simulink subsystem "ElectricMachine2"  (R2025b)
settings: Solver=VariableStepAuto  StartTime=0.0  StopTime=10.0  RelTol=1e-3
libraries: autolibmappedmotor x2
settings Model: ModifiedByFormat=The MathWorks, Inc.  Creator=The MathWorks, Inc.  LastModifiedBy=The MathWorks, Inc.
settings SolverCC: MaxZcPerStep=1.0
settings DebuggingCC: UnconnectedInputMsg=warning  UnconnectedOutputMsg=warning  UnconnectedLineMsg=warning
settings ModelReferenceCC: EnableRefExpFcnMdlSchedulingChecks=on
settings RTWCC: GPUComputeCapability=3.5  DLArmComputeVersion=19.05

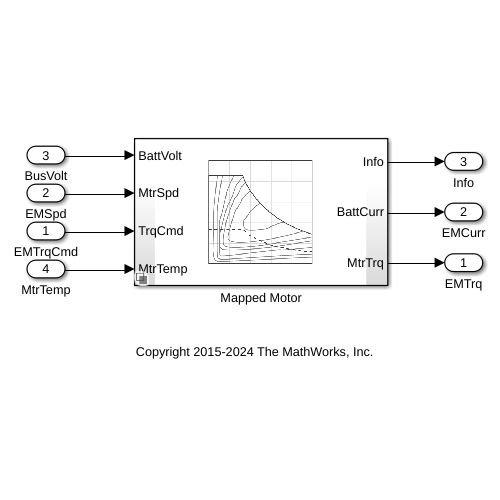
[thumbnail: Simulink's stored preview of the top-level diagram]
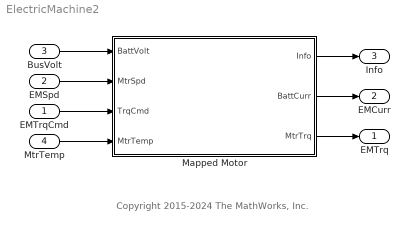
== system ElectricMachine2 ==
  note: Copyright 2015-2024 The MathWorks, Inc.
  EMTrqCmd : Inport
  EMSpd : Inport  Port=2
  BusVolt : Inport  Port=3
  MtrTemp : Inport  Port=4
  Mapped Motor : Subsystem  Variant=on  VariantControlMode=label  LabelModeActiveChoice=MappedMotorCalibrationImport
  EMTrq : Outport  VectorParamsAs1DForOutWhenUnconnected=off
  EMCurr : Outport  Port=2  VectorParamsAs1DForOutWhenUnconnected=off
  Info : Outport  Port=3
  wires:
  EMTrqCmd/1 -> Mapped Motor/3(TrqCmd)
  BusVolt/1 -> Mapped Motor/1(BattVolt)
  EMSpd/1 -> Mapped Motor/2(MtrSpd)
  Mapped Motor/2(BattCurr) -> EMCurr/1
  Mapped Motor/1(Info) -> Info/1
  Mapped Motor/3(MtrTrq) -> EMTrq/1
  MtrTemp/1 -> Mapped Motor/4(MtrTemp)

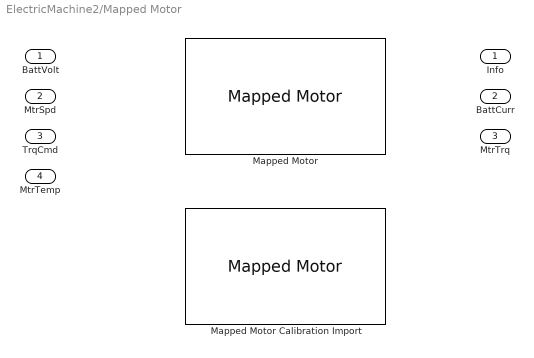
== system ElectricMachine2/Mapped Motor ==
  BattVolt : Inport
  MtrSpd : Inport  Port=2
  TrqCmd : Inport  Port=3
  MtrTemp : Inport  Port=4
  Mapped Motor : autolibmappedmotor/Mapped Motor  VariantControl=MappedMotor  w_Tmax_bp_ext=w_Tmax_bp  Tmax_w_V_ext=Tmax_w_V  w_Tmin_bp_ext=w_Tmin_bp  Tmin_w_V_ext=Tmin_w_V  port_config=Speed  param_by=Tabulated torque-speed envelope  w_t=PlntEM2Spd  T_t=PlntEM2Trq  torque_max=0.1  power_max=30  SpreadsheetTqLimitsFileName=MotorCalibrationImportData.xlsx  Tmax_w_V=PlntEM1MaxTqTbl  w_Tmax_bp=PlntEM1MaxTqSpdBpt  V_Tmax_bp=PlntEM1MaxTqVoltBpt  Tmin_w_V=PlntEM1MinTqTbl  w_Tmin_bp=PlntEM1MinTqSpdBpt  V_Tmin_bp=PlntEM1MinTqVoltBpt  Tc=PlntEM2TimeCnst  param_loss=Tabulated efficiency data  SpreadsheetLossFileName=MotorCalibrationImportData.xlsx  SpreadsheetEffFileName=MotorCalibrationImportData.xlsx  eff=100  w_eff=375  T_eff=0.08  Piron=0  Pbase=0  w_eff_bp=PlntEM2SpdEff  T_eff_bp=PlntEM2TrqEff  Temp_eff_bp=PlntEM1EffPwrLossTempBpt  V_eff_bp=PlntEM1EffPwrLossVoltBpt  losses_table=PlntEM2LossTbl  losses_table_3d=losses_table_3d  losses_table_4d=PlntEM1LossesTbl4d  efficiency_table=PlntEM2EffTbl  efficiency_table_3d=efficiency_table_3d  efficiency_table_4d=PlntEM1EffTbl4d  J=5e-6  b=1e-5  omega_o=0  T_t_extended=[47.7464829275686 52.0870722846203 57.2957795130823 63.6619772367581 71.6197243913529 81.8511135901176 95.4929658551372 114.591559026165 143.239448782706 190.985931710274 200 200 200 200 200 200 200 190.985931710274 143.239448782706 114.591559026165 95.4929658551372 81.8511135901176 71.6197243913529 63.6619772367581 57.2957795130823 52.0870722846203 47.7464829275686]  w_t_extended=[-628.318530717959 -575.958653158129 -523.598775598299 -471.238898038469 -418.879020478639 -366.519142918809 -314.159265358979 -261.799387799149 -209.43951023932 -157.07963267949 -149.999649206931 -104.71975511966 -52.3598775598299 0 52.3598775598299 104.71975511966 149.999649206931 157.07963267949 209.43951023932 261.799387799149 314.159265358979 366.519142918809 418.879020478639 471.238898038469 523.598775598299 575.958653158129 628.318530717959]  KLossIron=0  KLossCopper=0  x_w_eff_vec=[-628.318530717959 -575.958653158129 -523.598775598299 -471.238898038469 -418.879020478639 -366.519142918809 -314.159265358979 -261.799387799149 -209.43951023932 -157.07963267949 -149.999649206931 -104.71975511966 -52.3598775598299 0 52.3598775598299 104.71975511966 149.999649206931 157.07963267949 209.43951023932 261.799387799149 314.159265358979 366.519142918809 418.879020478639 471.238898038469 523.598775598299 575.958653158129 628.318530717959]  x_T_eff_vec=[-200 -180 -160 -140 -120 -100 -80 -60 -40 -20 0 20 40 60 80 100 120 140 160 180 200]  x_tmp_eff_vec=[233.15 293.15 373.15]  x_V_eff_vec=[233.15 293.15 373.15]  x_losses_mat=[9458.558526937 8512.7026742433 7566.8468215496 6620.9909688559 5675.1351161622 4729.2792634685 3783.4234107748 2837.5675580811 2485.6557259172 2045.68823954684 0 1759.29188601028 2261.94671058465 2638.93782901542 3518.58377202057 4398.22971502571 5277.87565803085 6157.52160103599 7037.16754404113 7916.81348704627 8796.45943005141;8670.34531635892 7803.31078472303 6936.27625308713 6069.24172145124 5202.20718981535 4335.17265817946 3468.13812654357 2601.10359490768 2003.3344457674 1875.21421958461 0 1612.68422884276 1843.06769010601 2419.02634326414 3225.36845768552 4031.7105721069 4838.05268652828 5644.39480094966 6450.73691537104 7257.07902979242 8063.4211442138;7882.13210578084 7093.91889520275 6305.70568462467 5517.49247404659 4729.2792634685 3941.06605289042 3152.85284231233 2364.63963173425 1821.21313251582 1704.74019962237 0 1466.07657167524 1675.51608191456 2199.11485751285 2932.15314335047 3665.19142918809 4398.22971502571 5131.26800086333 5864.30628670094 6597.34457253856 7330.38285837618;7093.91889520275 6384.52700568248 5675.1351161622 4965.74322664193 4256.35133712165 3546.95944760138 2837.5675580811 2128.17566856083 1864.2417944379 1534.26617966013 0 1319.46891450771 1696.46003293849 1979.20337176157 2638.93782901542 3298.67228626928 3958.40674352314 4618.14120077699 5277.87565803085 5937.61011528471 6597.34457253856;6305.70568462467 5675.1351161622 5044.56454769974 4413.99397923727 3783.4234107748 3152.85284231233 2522.28227384987 1891.7117053874 1657.10381727813 1363.7921596979 0 1172.86125734019 1507.9644737231 1759.29188601028 2345.72251468038 2932.15314335047 3518.58377202057 4105.01440069066 4691.44502936075 5277.87565803085 5864.30628670094;5517.49247404658 4965.74322664193 4413.99397923727 3862.24473183261 3310.49548442795 2758.74623702329 2549.69838552215 1912.27378914161 1628.97396852804 1396.26340159546 0 1172.86125734019 1466.07657167524 1759.29188601028 2345.72251468038 2565.63400043166 3078.76080051799 3591.88760060433 4105.01440069066 4618.14120077699 5131.26800086332;4729.2792634685 4256.35133712165 3783.4234107748 3310.49548442795 2837.5675580811 2731.81969877373 2485.6557259172 1864.2417944379 1713.59599286716 1379.23579913698 0 1130.97335529233 1507.9644737231 1696.46003293849 2261.94671058465 2513.27412287183 2638.93782901542 3078.760800518 3518.58377202057 3958.40674352314 4398.22971502571;5178.44942899416 4660.60448609474 3642.42626503164 3187.12298190269 2731.81969877373 2589.22471449708 2071.37977159766 1745.32925199433 1427.99666072263 1149.36316594749 0 942.477796076938 1256.63706143592 1570.7963267949 1884.95559215388 2356.19449019234 2513.27412287183 2932.15314335047 3351.03216382911 4241.15008234622 4712.38898038469;5711.98664289054 5140.78797860148 4569.58931431243 3257.94793705608 2792.52680319093 2327.10566932577 1861.68453546062 1713.59599286716 1363.7921596979 1047.1975511966 0 837.758040957278 1172.86125734019 1507.9644737231 1675.51608191456 2094.39510239319 2513.27412287183 2932.15314335047 4021.23859659494 4523.8934211693 5026.54824574367;5114.22059886711 4602.7985389804 4091.37647909369 2998.79298751753 2570.39398930074 2141.99499108395 1713.59599286716 1285.19699465037 1022.84411977342 785.398163397448 0 628.318530717959 879.645943005142 1130.97335529233 1507.9644737231 1884.95559215388 2261.94671058465 2638.93782901543 3518.58377202057 3958.40674352314 4398.22971502571;5714.27235074022 5142.8451156662 3906.96760725029 3418.596656344 2454.53971429523 2045.44976191269 1636.35980953016 1465.11285271886 976.741901812573 749.998246034654 0 599.998596827723 839.998035558812 1259.99705333822 1439.99663238654 1799.99579048317 2159.9949485798 2939.99312445584 3359.99214223525 4319.98989715961 4799.98877462179;4597.45266378994 4137.70739741095 3191.45920364677 2792.52680319093 2045.68823954684 1704.74019962237 1363.7921596979 1022.84411977342 797.864800911693 590.726823751927 0 460.766922526503 670.206432765823 879.645943005142 1172.86125734019 1466.07657167524 1759.29188601028 ...(+4852 chars)]  x_losses_mat_3d=cat(3,[2 2 2 2 2 2 2 2 2 2 2 2 2 2 2 2 2 2 2 2 2;2 2 2 2 2 2 2 2 2 2 2 2 2 2 2 2 2 2 2 2 2;2 2 2 2 2 2 2 2 2 2 2 2 2 2 2 2 2 2 2 2 2;2 2 2 2 2 2 2 2 2 2 2 2 2 2 2 2 2 2 2 2 2;2 2 2 2 2 2 2 2 2 2 2 2 2 2 2 2 2 2 2 2 2;2 2 2 2 2 2 2 2 2 2 2 2 2 2 2 2 2 2 2 2 2;2 2 2 2 2 2 2 2 2 2 2 2 2 2 2 2 2 2 2 2 2;2 2 2 2 2 2 2 2 2 2 2 2 2 2 2 2 2 2 2 2 2;2 2 2 2 2 2 2 2 2 2 2 2 2 2 2 2 2 2 2 2 2;2 2 2 2 2 2 2 2 2 2 2 2 2 2 2 2 2 2 2 2 2;2 2 2 2 2 2 2 2 2 2 2 2 2 2 2 2 2 2 2 2 2;2 2 2 2 2 2 2 2 2 2 2 2 2 2 2 2 2 2 2 2 2;2 2 2 2 2 2 2 2 2 2 2 2 2 2 2 2 2 2 2 2 2;2 2 2 2 2 2 2 2 2 2 2 2 2 2 2 2 2 2 2 2 2;2 2 2 2 2 2 2 2 2 2 2 2 2 2 2 2 2 2 2 2 2;2 2 2 2 2 2 2 2 2 2 2 2 2 2 2 2 2 2 2 2 2;2 2 2 2 2 2 2 2 2 2 2 2 2 2 2 2 2 2 2 2 2;2 2 2 2 2 2 2 2 2 2 2 2 2 2 2 2 2 2 2 2 2;2 2 2 2 2 2 2 2 2 2 2 2 2 2 2 2 2 2 2 2 2;2 2 2 2 2 2 2 2 2 2 2 2 2 2 2 2 2 2 2 2 2;2 2 2 2 2 2 2 2 2 2 2 2 2 2 2 2 2 2 2 2 2;2 2 2 2 2 2 2 2 2 2 2 2 2 2 2 2 2 2 2 2 2;2 2 2 2 2 2 2 2 2 2 2 2 2 2 2 2 2 2 2 2 2;2 2 2 2 2 2 2 2 2 2 2 2 2 2 2 2 2 2 2 2 2;2 2 2 2 2 2 2 2 2 2 2 2 2 2 2 2 2 2 2 2 2;2 2 2 2 2 2 2 2 2 2 2 2 2 2 2 2 2 2 2 2 2;2 2 2 2 2 2 2 2 2 2 2 2 2 2 2 2 2 2 2 2 2],[1.5 1.5 1.5 1.5 1.5 1.5 1.5 1.5 1.5 1.5 1.5 1.5 1.5 1.5 1.5 1.5 1.5 1.5 1.5 1.5 1.5;1.5 1.5 1.5 1.5 1.5 1.5 1.5 1.5 1.5 1.5 1.5 1.5 1.5 1.5 1.5 1.5 1.5 1.5 1.5 1.5 1.5;1.5 1.5 1.5 1.5 1.5 1.5 1.5 1.5 1.5 1.5 1.5 1.5 1.5 1.5 1.5 1.5 1.5 1.5 1.5 1.5 1.5;1.5 1.5 1.5 1.5 1.5 1.5 1.5 1.5 1.5 1.5 1.5 1.5 1.5 1.5 1.5 1.5 1.5 1.5 1.5 1.5 1.5;1.5 1.5 1.5 1.5 1.5 1.5 1.5 1.5 1.5 1.5 1.5 1.5 1.5 1.5 1.5 1.5 1.5 1.5 1.5 1.5 1.5;1.5 1.5 1.5 1.5 1.5 1.5 1.5 1.5 1.5 1.5 1.5 1.5 1.5 1.5 1.5 1.5 1.5 1.5 1.5 1.5 1.5;1.5 1.5 1.5 1.5 1.5 1.5 1.5 1.5 1.5 1.5 1.5 1.5 1.5 1.5 1.5 1.5 1.5 1.5 1.5 1.5 1.5;1.5 1.5 1.5 1.5 1.5 1.5 1.5 1.5 1.5 1.5 1.5 1.5 1.5 1.5 1.5 1.5 1.5 1.5 1.5 1.5 1.5;1.5 1.5 1.5 1.5 1.5 1.5 1.5 1.5 1.5 1.5 1.5 1.5 1.5 1.5 1.5 1.5 1.5 1.5 1.5 1.5 1.5;1.5 1.5 1.5 1.5 1.5 1.5 1.5 1.5 1.5 1.5 1.5 1.5 1.5 1.5 1.5 1.5 1.5 1.5 1.5 1.5 1.5;1.5 1.5 1.5 1.5 1.5 1.5 1.5 1.5 1.5 1.5 1.5 1.5 1.5 1.5 1.5 1.5 1.5 1.5 1.5 1.5 1.5;1.5 1.5 1.5 1.5 1.5 1.5 1.5 1.5 1.5 1.5 1.5 1.5 1.5 1.5 1.5 1.5 1.5 1.5 1.5 1.5 1.5;1.5 1.5 1.5 1.5 1.5 1.5 1.5 1.5 1.5 1.5 1.5 1.5 1.5 1.5 1.5 1.5 1.5 1.5 1.5 1.5 1.5;1.5 1.5 1.5 1.5 1.5 1.5 1.5 1.5 1.5 1.5 1.5 1.5 1.5 1.5 1.5 1.5 1.5 1.5 1.5 1.5 1.5;1.5 1.5 1.5 1.5 1.5 1.5 1.5 1.5 1.5 1.5 1.5 1.5 1.5 1.5 1.5 1.5 1.5 1.5 1.5 1.5 1.5;1.5 1.5 1.5 1.5 1.5 1.5 1.5 1.5 1.5 1.5 1.5 1.5 1.5 1.5 1.5 1.5 1.5 1.5 1.5 1.5 1.5;1.5 1.5 1.5 1.5 1.5 1.5 1.5 1.5 1.5 1.5 1.5 1.5 1.5 1.5 1.5 1.5 1.5 1.5 1.5 1.5 1.5;1.5 1.5 1.5 1.5 1.5 1.5 1.5 1.5 1.5 1.5 1.5 1.5 1.5 1.5 1.5 1.5 1.5 1.5 1.5 1.5 1.5;1.5 1.5 1.5 1.5 1.5 1.5 1.5 1.5 1.5 1.5 1.5 1.5 1.5 1.5 1.5 1.5 1.5 1.5 1.5 1.5 1.5;1.5 1.5 1.5 1.5 1.5 1.5 1.5 1.5 1.5 1.5 1.5 1.5 1.5 1.5 1.5 1.5 1.5 1.5 1.5 1.5 1.5;1.5 1.5 1.5 1.5 1.5 1.5 1.5 1.5 1.5 1.5 1.5 1.5 1.5 1.5 1.5 1.5 1.5 1.5 1.5 1.5 1.5;1.5 1.5 1.5 1.5 1.5 1.5 1.5 1.5 1.5 1.5 1.5 1.5 1.5 1.5 1.5 1.5 1.5 1.5 1.5 1.5 1.5;1.5 1.5 1.5 1.5 1.5 1.5 1.5 1.5 1.5 1.5 1.5 1.5 1.5 1.5 1.5 1.5 1.5 1.5 1.5 1.5 1.5;1.5 1.5 1.5 1.5 1.5 1.5 1.5 1.5 1.5 1.5 1.5 1.5 1.5 1.5 1.5 1.5 1.5 1.5 1.5 1.5 1.5;1.5 1.5 1.5 1.5 1.5 1.5 1.5 1.5 1.5 1.5 1.5 1.5 1.5 1.5 1.5 1.5 1.5 1.5 1.5 1.5 1.5;1.5 1.5 1.5 1.5 1.5 1.5 1.5 1.5 1.5 1.5 1.5 1.5 1.5 1.5 1.5 1.5 1.5 1.5 1.5 1.5 1.5;1.5 1.5 1.5 1.5 1.5 1.5 1.5 1.5 1.5 1.5 1.5 1.5 1.5 1.5 1.5 1.5 1.5 1.5 1.5 1.5 1.5],[1.9 1.9 1.9 1.9 1.9 1.9 1.9 1.9 1.9 1.9 1.9 1.9 1.9 1.9 1.9 1.9 1.9 1.9 1.9 1.9 1.9;1.9 1.9 1.9 1.9 1.9 1.9 1.9 1.9 1.9 1.9 1.9 1.9 1.9 1.9 1.9 1.9 1.9 1.9 1.9 1.9 1.9;1.9 1.9 1.9 1.9 1.9 1.9 1.9 1.9 1.9 1.9 1.9 1.9 1.9 1.9 1.9 1.9 1.9 1.9 1.9 1.9 1.9;1.9 1.9 1.9 1.9 1.9 1.9 1.9 1.9 1.9 1.9 1.9 1.9 1.9 1.9 1.9 1.9 1.9 1.9 1.9 1.9 1.9;1.9 1.9 1.9 1.9 1.9 1.9 1.9 1.9 1.9 1.9 1.9 1.9 1.9 1.9 1.9 1.9 1.9 1.9 1.9 1.9 1.9;1.9 1.9 1.9 1.9 1.9 1.9 1.9 1.9 1.9 1.9 1.9 1.9 1.9 1.9 1.9 1.9 1.9 1.9 1.9 1.9 1.9;1.9 1.9 1.9 1.9 1.9 1.9 1.9 1.9 1.9 1.9 1.9 1.9 1.9 1.9 1.9 1.9 1.9 1.9 1.9 1.9 1.9 ...(+1680 chars)])  x_losses_mat_4d=cat(4,cat(3,[1.5645 0.441 0.063 0.441 1.5645;1.7535 0.7245 0.252 0.7245 1.7535;2.3205 1.197 0.819 1.197 2.3205;3.255 2.1315 1.764 2.1315 3.255],[1.5645 0.441 0.063 0.441 1.5645;1.7535 0.7245 0.252 0.7245 1.7535;2.3205 1.197 0.819 1.197 2.3205;3.255 2.1315 1.764 2.1315 3.255],[1.5645 0.441 0.063 0.441 1.5645;1.7535 0.7245 0.252 0.7245 1.7535;2.3205 1.197 0.819 1.197 2.3205;3.255 2.1315 1.764 2.1315 3.255]),cat(3,[1.49 0.42 0.06 0.42 1.49;1.67 0.69 0.24 0.69 1.67;2.21 1.14 0.78 1.14 2.21;3.1 2.03 1.68 2.03 3.1],[1.49 0.42 0.06 0.42 1.49;1.67 0.69 0.24 0.69 1.67;2.21 1.14 0.78 1.14 2.21;3.1 2.03 1.68 2.03 3.1],[1.49 0.42 0.06 0.42 1.49;1.67 0.69 0.24 0.69 1.67;2.21 1.14 0.78 1.14 2.21;3.1 2.03 1.68 2.03 3.1]),cat(3,[1.5347 0.4326 0.0618 0.4326 1.5347;1.7201 0.7107 0.2472 0.7107 1.7201;2.2763 1.1742 0.8034 1.1742 2.2763;3.193 2.0909 1.7304 2.0909 3.193],[1.5347 0.4326 0.0618 0.4326 1.5347;1.7201 0.7107 0.2472 0.7107 1.7201;2.2763 1.1742 0.8034 1.1742 2.2763;3.193 2.0909 1.7304 2.0909 3.193],[1.5347 0.4326 0.0618 0.4326 1.5347;1.7201 0.7107 0.2472 0.7107 1.7201;2.2763 1.1742 0.8034 1.1742 2.2763;3.193 2.0909 1.7304 2.0909 3.193]))  CalLossMapData={'BaseCageProjectFileName','';'BaseMbcProjectFileName','';'TaskName','Calibrate Motor Loss Map';'ChildTasks',{{'DataName','';'TaskName','Import Loss Data'},{'TaskName','Generate Response Models'},{'TaskName','Generate Calibration'},{'TaskName','Update Block Parameters'}}}  CalLossWithTempMapData={}  aMode=6  RefBlkName='autolibmappedmotor/Mapped Motor'
  Mapped Motor Calibration Import : autolibmappedmotor/Mapped Motor  VariantControl=MappedMotorCalibrationImport  w_Tmax_bp_ext=w_Tmax_bp  Tmax_w_V_ext=Tmax_w_V  w_Tmin_bp_ext=w_Tmin_bp  Tmin_w_V_ext=Tmin_w_V  port_config=Speed  param_by=Tabulated torque-speed-voltage envelope  w_t=PlntEM1Spd  T_t=PlntEM1Trq  torque_max=0.1  power_max=30  SpreadsheetTqLimitsFileName=MotorCalibrationImportData.xlsx  Tmax_w_V=PlntEM2MaxTqTbl  w_Tmax_bp=PlntEM2MaxTqSpdBpt  V_Tmax_bp=PlntEM2MaxTqVoltBpt  Tmin_w_V=PlntEM2MinTqTbl  w_Tmin_bp=PlntEM2MinTqSpdBpt  V_Tmin_bp=PlntEM2MinTqVoltBpt  Tc=PlntEM2TimeCnst  param_loss=Tabulated loss data with temperature and voltage  SpreadsheetLossFileName=MotorCalibrationImportData.xlsx  SpreadsheetEffFileName=MotorCalibrationImportData.xlsx  eff=100  w_eff=375  T_eff=0.08  Piron=0  Pbase=0  w_eff_bp=PlntEM2EffPwrLossSpdBpt  T_eff_bp=PlntEM2EffPwrLossTrqBpt  Temp_eff_bp=PlntEM2EffPwrLossTempBpt  V_eff_bp=PlntEM2EffPwrLossVoltBpt  losses_table=PlntEM1TrqLossTbl  losses_table_3d=losses_table_3d  losses_table_4d=PlntEM2LossesTbl4d  efficiency_table=PlntEM1EffTbl  efficiency_table_3d=efficiency_table_3d  efficiency_table_4d=PlntEM2EffTbl4d  J=5e-6  b=1e-5  omega_o=0  T_t_extended=[47.7464829275686 52.0870722846203 57.2957795130823 63.6619772367581 71.6197243913529 81.8511135901176 95.4929658551372 114.591559026165 143.239448782706 190.985931710274 200 200 200 200 200 200 200 190.985931710274 143.239448782706 114.591559026165 95.4929658551372 81.8511135901176 71.6197243913529 63.6619772367581 57.2957795130823 52.0870722846203 47.7464829275686]  w_t_extended=[-628.318530717959 -575.958653158129 -523.598775598299 -471.238898038469 -418.879020478639 -366.519142918809 -314.159265358979 -261.799387799149 -209.43951023932 -157.07963267949 -149.999649206931 -104.71975511966 -52.3598775598299 0 52.3598775598299 104.71975511966 149.999649206931 157.07963267949 209.43951023932 261.799387799149 314.159265358979 366.519142918809 418.879020478639 471.238898038469 523.598775598299 575.958653158129 628.318530717959]  KLossIron=0  KLossCopper=0  x_w_eff_vec=[-628.318530717959 -575.958653158129 -523.598775598299 -471.238898038469 -418.879020478639 -366.519142918809 -314.159265358979 -261.799387799149 -209.43951023932 -157.07963267949 -149.999649206931 -104.71975511966 -52.3598775598299 0 52.3598775598299 104.71975511966 149.999649206931 157.07963267949 209.43951023932 261.799387799149 314.159265358979 366.519142918809 418.879020478639 471.238898038469 523.598775598299 575.958653158129 628.318530717959]  x_T_eff_vec=[-200 -180 -160 -140 -120 -100 -80 -60 -40 -20 0 20 40 60 80 100 120 140 160 180 200]  x_tmp_eff_vec=[233.15 293.15 373.15]  x_V_eff_vec=[233.15 293.15 373.15]  x_losses_mat=[9458.558526937 8512.7026742433 7566.8468215496 6620.9909688559 5675.1351161622 4729.2792634685 3783.4234107748 2837.5675580811 2485.6557259172 2045.68823954684 0 1759.29188601028 2261.94671058465 2638.93782901542 3518.58377202057 4398.22971502571 5277.87565803085 6157.52160103599 7037.16754404113 7916.81348704627 8796.45943005141;8670.34531635892 7803.31078472303 6936.27625308713 6069.24172145124 5202.20718981535 4335.17265817946 3468.13812654357 2601.10359490768 2003.3344457674 1875.21421958461 0 1612.68422884276 1843.06769010601 2419.02634326414 3225.36845768552 4031.7105721069 4838.05268652828 5644.39480094966 6450.73691537104 7257.07902979242 8063.4211442138;7882.13210578084 7093.91889520275 6305.70568462467 5517.49247404659 4729.2792634685 3941.06605289042 3152.85284231233 2364.63963173425 1821.21313251582 1704.74019962237 0 1466.07657167524 1675.51608191456 2199.11485751285 2932.15314335047 3665.19142918809 4398.22971502571 5131.26800086333 5864.30628670094 6597.34457253856 7330.38285837618;7093.91889520275 6384.52700568248 5675.1351161622 4965.74322664193 4256.35133712165 3546.95944760138 2837.5675580811 2128.17566856083 1864.2417944379 1534.26617966013 0 1319.46891450771 1696.46003293849 1979.20337176157 2638.93782901542 3298.67228626928 3958.40674352314 4618.14120077699 5277.87565803085 5937.61011528471 6597.34457253856;6305.70568462467 5675.1351161622 5044.56454769974 4413.99397923727 3783.4234107748 3152.85284231233 2522.28227384987 1891.7117053874 1657.10381727813 1363.7921596979 0 1172.86125734019 1507.9644737231 1759.29188601028 2345.72251468038 2932.15314335047 3518.58377202057 4105.01440069066 4691.44502936075 5277.87565803085 5864.30628670094;5517.49247404658 4965.74322664193 4413.99397923727 3862.24473183261 3310.49548442795 2758.74623702329 2549.69838552215 1912.27378914161 1628.97396852804 1396.26340159546 0 1172.86125734019 1466.07657167524 1759.29188601028 2345.72251468038 2565.63400043166 3078.76080051799 3591.88760060433 4105.01440069066 4618.14120077699 5131.26800086332;4729.2792634685 4256.35133712165 3783.4234107748 3310.49548442795 2837.5675580811 2731.81969877373 2485.6557259172 1864.2417944379 1713.59599286716 1379.23579913698 0 1130.97335529233 1507.9644737231 1696.46003293849 2261.94671058465 2513.27412287183 2638.93782901542 3078.760800518 3518.58377202057 3958.40674352314 4398.22971502571;5178.44942899416 4660.60448609474 3642.42626503164 3187.12298190269 2731.81969877373 2589.22471449708 2071.37977159766 1745.32925199433 1427.99666072263 1149.36316594749 0 942.477796076938 1256.63706143592 1570.7963267949 1884.95559215388 2356.19449019234 2513.27412287183 2932.15314335047 3351.03216382911 4241.15008234622 4712.38898038469;5711.98664289054 5140.78797860148 4569.58931431243 3257.94793705608 2792.52680319093 2327.10566932577 1861.68453546062 1713.59599286716 1363.7921596979 1047.1975511966 0 837.758040957278 1172.86125734019 1507.9644737231 1675.51608191456 2094.39510239319 2513.27412287183 2932.15314335047 4021.23859659494 4523.8934211693 5026.54824574367;5114.22059886711 4602.7985389804 4091.37647909369 2998.79298751753 2570.39398930074 2141.99499108395 1713.59599286716 1285.19699465037 1022.84411977342 785.398163397448 0 628.318530717959 879.645943005142 1130.97335529233 1507.9644737231 1884.95559215388 2261.94671058465 2638.93782901543 3518.58377202057 3958.40674352314 4398.22971502571;5714.27235074022 5142.8451156662 3906.96760725029 3418.596656344 2454.53971429523 2045.44976191269 1636.35980953016 1465.11285271886 976.741901812573 749.998246034654 0 599.998596827723 839.998035558812 1259.99705333822 1439.99663238654 1799.99579048317 2159.9949485798 2939.99312445584 3359.99214223525 4319.98989715961 4799.98877462179;4597.45266378994 4137.70739741095 3191.45920364677 2792.52680319093 2045.68823954684 1704.74019962237 1363.7921596979 1022.84411977342 797.864800911693 590.726823751927 0 460.766922526503 670.206432765823 879.645943005142 1172.86125734019 1466.07657167524 1759.29188601028 ...(+4852 chars)]  x_losses_mat_3d=cat(3,[2 2 2 2 2 2 2 2 2 2 2 2 2 2 2 2 2 2 2 2 2;2 2 2 2 2 2 2 2 2 2 2 2 2 2 2 2 2 2 2 2 2;2 2 2 2 2 2 2 2 2 2 2 2 2 2 2 2 2 2 2 2 2;2 2 2 2 2 2 2 2 2 2 2 2 2 2 2 2 2 2 2 2 2;2 2 2 2 2 2 2 2 2 2 2 2 2 2 2 2 2 2 2 2 2;2 2 2 2 2 2 2 2 2 2 2 2 2 2 2 2 2 2 2 2 2;2 2 2 2 2 2 2 2 2 2 2 2 2 2 2 2 2 2 2 2 2;2 2 2 2 2 2 2 2 2 2 2 2 2 2 2 2 2 2 2 2 2;2 2 2 2 2 2 2 2 2 2 2 2 2 2 2 2 2 2 2 2 2;2 2 2 2 2 2 2 2 2 2 2 2 2 2 2 2 2 2 2 2 2;2 2 2 2 2 2 2 2 2 2 2 2 2 2 2 2 2 2 2 2 2;2 2 2 2 2 2 2 2 2 2 2 2 2 2 2 2 2 2 2 2 2;2 2 2 2 2 2 2 2 2 2 2 2 2 2 2 2 2 2 2 2 2;2 2 2 2 2 2 2 2 2 2 2 2 2 2 2 2 2 2 2 2 2;2 2 2 2 2 2 2 2 2 2 2 2 2 2 2 2 2 2 2 2 2;2 2 2 2 2 2 2 2 2 2 2 2 2 2 2 2 2 2 2 2 2;2 2 2 2 2 2 2 2 2 2 2 2 2 2 2 2 2 2 2 2 2;2 2 2 2 2 2 2 2 2 2 2 2 2 2 2 2 2 2 2 2 2;2 2 2 2 2 2 2 2 2 2 2 2 2 2 2 2 2 2 2 2 2;2 2 2 2 2 2 2 2 2 2 2 2 2 2 2 2 2 2 2 2 2;2 2 2 2 2 2 2 2 2 2 2 2 2 2 2 2 2 2 2 2 2;2 2 2 2 2 2 2 2 2 2 2 2 2 2 2 2 2 2 2 2 2;2 2 2 2 2 2 2 2 2 2 2 2 2 2 2 2 2 2 2 2 2;2 2 2 2 2 2 2 2 2 2 2 2 2 2 2 2 2 2 2 2 2;2 2 2 2 2 2 2 2 2 2 2 2 2 2 2 2 2 2 2 2 2;2 2 2 2 2 2 2 2 2 2 2 2 2 2 2 2 2 2 2 2 2;2 2 2 2 2 2 2 2 2 2 2 2 2 2 2 2 2 2 2 2 2],[1.5 1.5 1.5 1.5 1.5 1.5 1.5 1.5 1.5 1.5 1.5 1.5 1.5 1.5 1.5 1.5 1.5 1.5 1.5 1.5 1.5;1.5 1.5 1.5 1.5 1.5 1.5 1.5 1.5 1.5 1.5 1.5 1.5 1.5 1.5 1.5 1.5 1.5 1.5 1.5 1.5 1.5;1.5 1.5 1.5 1.5 1.5 1.5 1.5 1.5 1.5 1.5 1.5 1.5 1.5 1.5 1.5 1.5 1.5 1.5 1.5 1.5 1.5;1.5 1.5 1.5 1.5 1.5 1.5 1.5 1.5 1.5 1.5 1.5 1.5 1.5 1.5 1.5 1.5 1.5 1.5 1.5 1.5 1.5;1.5 1.5 1.5 1.5 1.5 1.5 1.5 1.5 1.5 1.5 1.5 1.5 1.5 1.5 1.5 1.5 1.5 1.5 1.5 1.5 1.5;1.5 1.5 1.5 1.5 1.5 1.5 1.5 1.5 1.5 1.5 1.5 1.5 1.5 1.5 1.5 1.5 1.5 1.5 1.5 1.5 1.5;1.5 1.5 1.5 1.5 1.5 1.5 1.5 1.5 1.5 1.5 1.5 1.5 1.5 1.5 1.5 1.5 1.5 1.5 1.5 1.5 1.5;1.5 1.5 1.5 1.5 1.5 1.5 1.5 1.5 1.5 1.5 1.5 1.5 1.5 1.5 1.5 1.5 1.5 1.5 1.5 1.5 1.5;1.5 1.5 1.5 1.5 1.5 1.5 1.5 1.5 1.5 1.5 1.5 1.5 1.5 1.5 1.5 1.5 1.5 1.5 1.5 1.5 1.5;1.5 1.5 1.5 1.5 1.5 1.5 1.5 1.5 1.5 1.5 1.5 1.5 1.5 1.5 1.5 1.5 1.5 1.5 1.5 1.5 1.5;1.5 1.5 1.5 1.5 1.5 1.5 1.5 1.5 1.5 1.5 1.5 1.5 1.5 1.5 1.5 1.5 1.5 1.5 1.5 1.5 1.5;1.5 1.5 1.5 1.5 1.5 1.5 1.5 1.5 1.5 1.5 1.5 1.5 1.5 1.5 1.5 1.5 1.5 1.5 1.5 1.5 1.5;1.5 1.5 1.5 1.5 1.5 1.5 1.5 1.5 1.5 1.5 1.5 1.5 1.5 1.5 1.5 1.5 1.5 1.5 1.5 1.5 1.5;1.5 1.5 1.5 1.5 1.5 1.5 1.5 1.5 1.5 1.5 1.5 1.5 1.5 1.5 1.5 1.5 1.5 1.5 1.5 1.5 1.5;1.5 1.5 1.5 1.5 1.5 1.5 1.5 1.5 1.5 1.5 1.5 1.5 1.5 1.5 1.5 1.5 1.5 1.5 1.5 1.5 1.5;1.5 1.5 1.5 1.5 1.5 1.5 1.5 1.5 1.5 1.5 1.5 1.5 1.5 1.5 1.5 1.5 1.5 1.5 1.5 1.5 1.5;1.5 1.5 1.5 1.5 1.5 1.5 1.5 1.5 1.5 1.5 1.5 1.5 1.5 1.5 1.5 1.5 1.5 1.5 1.5 1.5 1.5;1.5 1.5 1.5 1.5 1.5 1.5 1.5 1.5 1.5 1.5 1.5 1.5 1.5 1.5 1.5 1.5 1.5 1.5 1.5 1.5 1.5;1.5 1.5 1.5 1.5 1.5 1.5 1.5 1.5 1.5 1.5 1.5 1.5 1.5 1.5 1.5 1.5 1.5 1.5 1.5 1.5 1.5;1.5 1.5 1.5 1.5 1.5 1.5 1.5 1.5 1.5 1.5 1.5 1.5 1.5 1.5 1.5 1.5 1.5 1.5 1.5 1.5 1.5;1.5 1.5 1.5 1.5 1.5 1.5 1.5 1.5 1.5 1.5 1.5 1.5 1.5 1.5 1.5 1.5 1.5 1.5 1.5 1.5 1.5;1.5 1.5 1.5 1.5 1.5 1.5 1.5 1.5 1.5 1.5 1.5 1.5 1.5 1.5 1.5 1.5 1.5 1.5 1.5 1.5 1.5;1.5 1.5 1.5 1.5 1.5 1.5 1.5 1.5 1.5 1.5 1.5 1.5 1.5 1.5 1.5 1.5 1.5 1.5 1.5 1.5 1.5;1.5 1.5 1.5 1.5 1.5 1.5 1.5 1.5 1.5 1.5 1.5 1.5 1.5 1.5 1.5 1.5 1.5 1.5 1.5 1.5 1.5;1.5 1.5 1.5 1.5 1.5 1.5 1.5 1.5 1.5 1.5 1.5 1.5 1.5 1.5 1.5 1.5 1.5 1.5 1.5 1.5 1.5;1.5 1.5 1.5 1.5 1.5 1.5 1.5 1.5 1.5 1.5 1.5 1.5 1.5 1.5 1.5 1.5 1.5 1.5 1.5 1.5 1.5;1.5 1.5 1.5 1.5 1.5 1.5 1.5 1.5 1.5 1.5 1.5 1.5 1.5 1.5 1.5 1.5 1.5 1.5 1.5 1.5 1.5],[1.9 1.9 1.9 1.9 1.9 1.9 1.9 1.9 1.9 1.9 1.9 1.9 1.9 1.9 1.9 1.9 1.9 1.9 1.9 1.9 1.9;1.9 1.9 1.9 1.9 1.9 1.9 1.9 1.9 1.9 1.9 1.9 1.9 1.9 1.9 1.9 1.9 1.9 1.9 1.9 1.9 1.9;1.9 1.9 1.9 1.9 1.9 1.9 1.9 1.9 1.9 1.9 1.9 1.9 1.9 1.9 1.9 1.9 1.9 1.9 1.9 1.9 1.9;1.9 1.9 1.9 1.9 1.9 1.9 1.9 1.9 1.9 1.9 1.9 1.9 1.9 1.9 1.9 1.9 1.9 1.9 1.9 1.9 1.9;1.9 1.9 1.9 1.9 1.9 1.9 1.9 1.9 1.9 1.9 1.9 1.9 1.9 1.9 1.9 1.9 1.9 1.9 1.9 1.9 1.9;1.9 1.9 1.9 1.9 1.9 1.9 1.9 1.9 1.9 1.9 1.9 1.9 1.9 1.9 1.9 1.9 1.9 1.9 1.9 1.9 1.9;1.9 1.9 1.9 1.9 1.9 1.9 1.9 1.9 1.9 1.9 1.9 1.9 1.9 1.9 1.9 1.9 1.9 1.9 1.9 1.9 1.9 ...(+1680 chars)])  x_losses_mat_4d=cat(4,cat(3,[1.5645 0.441 0.063 0.441 1.5645;1.7535 0.7245 0.252 0.7245 1.7535;2.3205 1.197 0.819 1.197 2.3205;3.255 2.1315 1.764 2.1315 3.255],[1.5645 0.441 0.063 0.441 1.5645;1.7535 0.7245 0.252 0.7245 1.7535;2.3205 1.197 0.819 1.197 2.3205;3.255 2.1315 1.764 2.1315 3.255],[1.5645 0.441 0.063 0.441 1.5645;1.7535 0.7245 0.252 0.7245 1.7535;2.3205 1.197 0.819 1.197 2.3205;3.255 2.1315 1.764 2.1315 3.255]),cat(3,[1.49 0.42 0.06 0.42 1.49;1.67 0.69 0.24 0.69 1.67;2.21 1.14 0.78 1.14 2.21;3.1 2.03 1.68 2.03 3.1],[1.49 0.42 0.06 0.42 1.49;1.67 0.69 0.24 0.69 1.67;2.21 1.14 0.78 1.14 2.21;3.1 2.03 1.68 2.03 3.1],[1.49 0.42 0.06 0.42 1.49;1.67 0.69 0.24 0.69 1.67;2.21 1.14 0.78 1.14 2.21;3.1 2.03 1.68 2.03 3.1]),cat(3,[1.5347 0.4326 0.0618 0.4326 1.5347;1.7201 0.7107 0.2472 0.7107 1.7201;2.2763 1.1742 0.8034 1.1742 2.2763;3.193 2.0909 1.7304 2.0909 3.193],[1.5347 0.4326 0.0618 0.4326 1.5347;1.7201 0.7107 0.2472 0.7107 1.7201;2.2763 1.1742 0.8034 1.1742 2.2763;3.193 2.0909 1.7304 2.0909 3.193],[1.5347 0.4326 0.0618 0.4326 1.5347;1.7201 0.7107 0.2472 0.7107 1.7201;2.2763 1.1742 0.8034 1.1742 2.2763;3.193 2.0909 1.7304 2.0909 3.193]))  CalLossMapData={'BaseCageProjectFileName','';'BaseMbcProjectFileName','';'TaskName','Calibrate Motor Loss Map';'ChildTasks',{{'DataName','';'TaskName','Import Loss Data'},{'TaskName','Generate Response Models'},{'TaskName','Generate Calibration'},{'TaskName','Update Block Parameters'}}}  CalLossWithTempMapData={}  aMode=6  RefBlkName='autolibmappedmotor/Mapped Motor'
  Info : Outport
  BattCurr : Outport  Port=2  VectorParamsAs1DForOutWhenUnconnected=off
  MtrTrq : Outport  Port=3  VectorParamsAs1DForOutWhenUnconnected=off
